simulink model "gazebo_cosim_test"  (R2019b)
settings: Solver=VariableStepAuto  StartTime=0.0  StopTime=4.3  RelTol=1e-3
undefined symbols (not defined in the file or in its folder): box, duration, force_type, fz, link, link_name, model_name, torque_type
libraries: robotgazebolib x5
settings Model: DataDictionary=performCoSimulationWithGazeboDD.sldd  Creator=The MathWorks, Inc.  LastModifiedBy=darrahts
settings DebuggingCC: SymbolicDimsDataTypeCodeGenerationDiagnostic=none

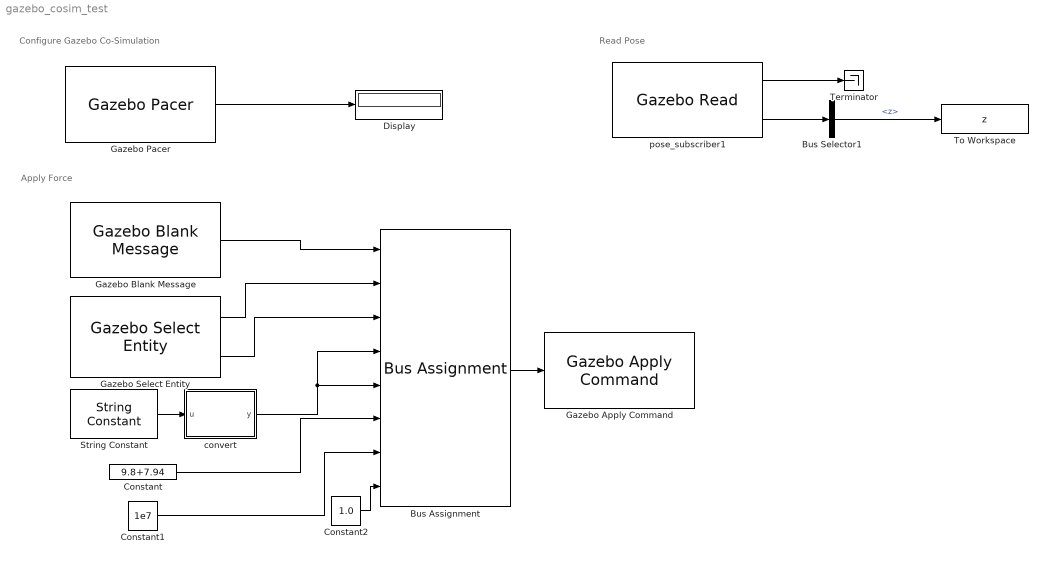
== system gazebo_cosim_test ==
  note: Read Pose
  note: Configure Gazebo Co-Simulation
  note: Apply Force
  Bus Assignment : BusAssignment  AssignedSignals=model_name,link_name,force_type,torque_type,fz,duration.nano_seconds,duration.seconds
  Bus Selector1 : BusSelector  OutputSignals=position.z
  Constant : Constant  Value=9.8+7.94
  Constant1 : Constant  Value=1e7
  Constant2 : Constant  Value=1.0
  Display : Display
  Gazebo Apply Command : robotgazebolib/Gazebo Apply Command  cmdType=ApplyLinkWrench  sampleTime=s
      settings: SourceProductName=Robotics System Toolbox  SourceProductBaseCode=RO
  Gazebo Blank Message : robotgazebolib/Gazebo Blank Message  msgType=ApplyLinkWrench  sampleTime=s  busName='Gazebo_SL_Bus_gazebo_msgs_ApplyLinkWrench'
      settings: SourceProductName=Robotics System Toolbox  SourceProductBaseCode=RO
  Gazebo Pacer : robotgazebolib/Gazebo Pacer  ResetBehavior=Reset Gazebo simulation time and scene  SampleTime=0.001
      settings: SourceProductName=Robotics System Toolbox  SourceProductBaseCode=RO
  Gazebo Select Entity : robotgazebolib/Gazebo Select Entity  modelElemName=box/link  outputArraySize=128  OutputLabel=Link  SelectType=Link
      settings: SourceProductName=Robotics System Toolbox  SourceProductBaseCode=RO
  String Constant : StringConstant  String="\"SET\""
  Terminator : Terminator
  To Workspace : ToWorkspace  VariableName=z  SaveFormat=Timeseries  SampleTime=-1
  convert : MATLAB Function  TreatAsAtomicUnit=on
  pose_subscriber1 : robotgazebolib/Gazebo Read  topicSource=From Gazebo  topic=/gazebo/ground_truth/world_pose/box/link  messageType=gazebo_msgs/Pose  sampleTime=s
      settings: SourceProductName=Robotics System Toolbox  SourceProductBaseCode=RO
  wires:
  Gazebo Pacer/1 -> Display/1
  Gazebo Blank Message/1 -> Bus Assignment/1
  Bus Assignment/1 -> Gazebo Apply Command/1
  Gazebo Select Entity/1 -> Bus Assignment/2
  Gazebo Select Entity/2 -> Bus Assignment/3
  String Constant/1 -> convert/1(u)
  convert/1(y) -> Bus Assignment/5, Bus Assignment/4
  Constant1/1 -> Bus Assignment/7
  Constant/1 -> Bus Assignment/6
  Constant2/1 -> Bus Assignment/8
  Bus Selector1/1 -> To Workspace/1  "<z>"
  pose_subscriber1/1 -> Terminator/1
  pose_subscriber1/2 -> Bus Selector1/1

== matlab function gazebo_cosim_test/convert ==
  data: u input; y output size=128
function y = convertStringToUInt8VarSize(u)

y = uint8(convertStringsToChars(u))';
